simulink model "test"  (R2020a)
settings: Solver=FixedStepAuto  StartTime=0.0  StopTime=inf  FixedStep=.001  RelTol=1e-3  EnableMultiTasking=on
libraries: GPIO_Lib x2, STM32_Config_Lib x1, USART_Lib x1
settings Model: Creator=brunj  LastModifiedBy=tuziz
settings DataIOCC: LimitDataPoints=on  SaveFormat=Array  ReturnWorkspaceOutputs=off
settings OptimizationCC: DefaultParameterBehavior=Inlined  PassReuseOutputArgsAs=Individual arguments  LifeSpan=1  EfficientTunableParamExpr=on
settings DebuggingCC: UnderspecifiedInitializationDetection=Classic  MergeDetectMultiDrivingBlocksExec=none  SolverPrmCheckMsg=warning  AllowSymbolicDim=off  StrictBusMsg=ErrorOnBusTreatedAsVector  SFUnexpectedBacktrackingDiag=warning  SFNoUnconditionalDefaultTransitionDiag=warning  SFUndirectedBroadcastEventsDiag=error  SFExecutionAtInitializationDiag=none  ArithmeticOperatorsInVariantConditions=warning
settings HardwareCC: ProdBitPerPointer=32  ProdBitPerSizeT=32  ProdBitPerPtrDiffT=32  ProdLargestAtomicInteger=Integer  ProdWordSize=32  ProdHWDeviceType=STMicroelectronics->STM32 32-bit Cortex-M
settings ModelReferenceCC: PropagateSignalLabelsOutOfModel=off
settings SFSimCC: SimUseLocalCustomCode=off  CompileTimeRecursionLimit=0  EnableRuntimeRecursion=off  MATLABDynamicMemAlloc=off  CustomCodeUndefinedFunction=UseInterfaceOnly
settings RTWCC: Description=stm32 (Embedded Target)  SystemTargetFile=stm32.tlc  TemplateMakefile=stm32.tmf  RTWUseLocalCustomCode=off  IncludeHyperlinkInReport=on
settings CodeAppCC: IgnoreCustomStorageClasses=off  CustomSymbolStrType=$N$R$M  SimulinkBlockComments=off
settings STFCustomTargetCC: ParMdlRefBuildCompliant=on  IncludeMdlTerminateFcn=off  CombineOutputUpdateFcns=on  ERTCustomFileBanners=on  SupportNonFinite=off  SupportComplex=off  SupportContinuousTime=off  SupportNonInlinedSFcns=off  RemoveResetFunc=on  ParenthesesLevel=Maximum  CastingMode=Standards  MATLABClassNameForMDSCustomization=Simulink.SoftwareTarget.ERTCustomization  SystemTargetFile=stm32.tlc
settings ERTTargetCC: MultiwordLength=2048  CompOptLevelCompliant=off  ConcurrentExecutionCompliant=off  IncludeMdlTerminateFcn=off  SupportNonFinite=off  SupportComplex=off  ParenthesesLevel=Maximum  CastingMode=Standards  ModelStepFunctionPrototypeControlCompliant=off  CPPClassGenCompliant=off  UseToolchainInfoCompliant=off  ExtModeTransport=1  ExtModeStaticAllocSize=256  ExtModeMexArgs=0,1,115200,10  InlinedParameterPlacement=NonHierarchical  ERTSrcFileBannerTemplate=sourceFileTemplate.cgt  ERTHdrFileBannerTemplate=sourceFileTemplate.cgt  ERTDataSrcFileTemplate=sourceFileTemplate.cgt  ERTDataHdrFileTemplate=sourceFileTemplate.cgt  ERTCustomFileTemplate=customRoutineProcess.tlc  ConvertIfToSwitch=off  SuppressUnreachableDefaultCases=off  EnableSignedLeftShifts=off  EnableSignedRightShifts=off
settings ConfigComp: CovMetricSettings=dw  CovHtmlReporting=on  CovSaveCumulativeToWorkspaceVar=on  CovSaveSingleToWorkspaceVar=on  CovExternalEMLEnable=off  CovSFcnEnable=off

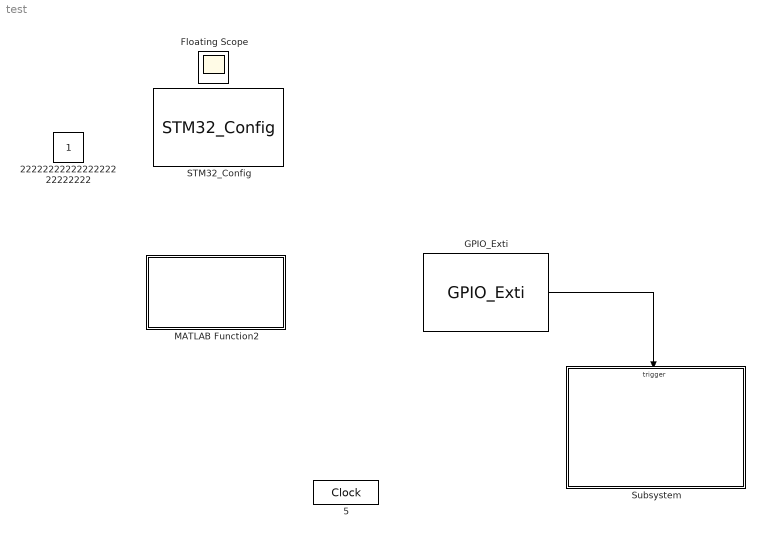
== system test ==
  GPIO_Exti : GPIO_Lib/GPIO_Exti  Port_name=GPIOE  Pin_0=on  Pin_1=off  Pin_2=off  Pin_3=off  Pin_4=off  Pin_5=off  Pin_6=off  Pin_7=off  Pin_8=off  Pin_9=off  Pin_10=off  Pin_11=off  Pin_12=off  Pin_13=off  Pin_14=off  Pin_15=off  PinList=GPIOE0
      settings: SourceProductName=Target Support Package - STM32 Adapter
  MATLAB Function2 : MATLAB Function  Priority=0  TreatAsAtomicUnit=on
  STM32_Config : STM32_Config_Lib/STM32_Config  Priority=0  Project_Path=.\  Config_File=test.ioc  MCU_Name=STM32F407VGTx
      settings: SourceProductName=Target Support Package - STM32 Adapter
  Subsystem : Subsystem
  2222222222222222222222222 : Constant  IOType=siggen
  5 : DigitalClock  IOType=siggen
  Floating Scope : Scope
  wires:
  GPIO_Exti/1 -> Subsystem/Trigger

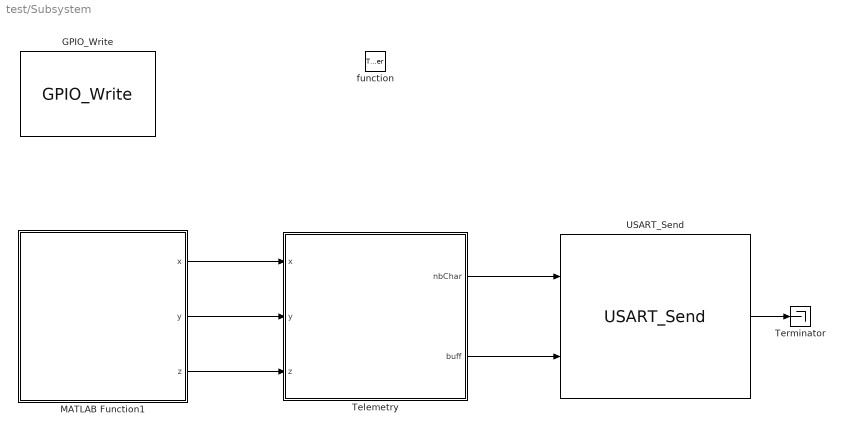
== system test/Subsystem ==
  function : TriggerPort  TriggerType=function-call  VariantControl=Variant
  GPIO_Write : GPIO_Lib/GPIO_Write  Port_name=GPIOD  Pin0=off  Toggle_Pin0=off  Pin1=off  Toggle_Pin1=off  Pin2=off  Toggle_Pin2=off  Pin3=off  Toggle_Pin3=off  Pin4=off  Toggle_Pin4=off  Pin5=off  Toggle_Pin5=off  Pin6=off  Toggle_Pin6=off  Pin7=off  Toggle_Pin7=off  Pin8=off  Toggle_Pin8=off  Pin9=off  Toggle_Pin9=off  Pin10=off  Toggle_Pin10=off  Pin11=off  Toggle_Pin11=off  Pin12=on  Toggle_Pin12=on  Pin13=off  Toggle_Pin13=off  Pin14=off  Toggle_Pin14=off  Pin15=off  Toggle_Pin15=off  PinList="GPIOD12  13  14  15GPIOE3"
      settings: SourceProductName=Target Support Package - STM32 Adapter
  MATLAB Function1 : MATLAB Function  Priority=0  TreatAsAtomicUnit=on
  Telemetry : MATLAB Function  TreatAsAtomicUnit=on
  Terminator : Terminator
  USART_Send : USART_Lib/USART_Send  USART_name=USART3  Buff_size=22  nbUsart=1  usartMode=Asynchronous  usartDma_Rx=off  usartDma_Tx=off  usartIt=on
      settings: SourceProductName=Target Support Package - STM32 Adapter
  wires:
  USART_Send/1 -> Terminator/1
  MATLAB Function1/2(y) -> Telemetry/2(y)
  Telemetry/1(nbChar) -> USART_Send/1
  Telemetry/2(buff) -> USART_Send/2
  MATLAB Function1/1(x) -> Telemetry/1(x)
  MATLAB Function1/3(z) -> Telemetry/3(z)

== matlab function test/MATLAB Function2 ==
function LIS302_Init()
if coder.target('Sfun')
    % Executing in MATLAB, Buff is null
else
    coder.cinclude('LIS3DSH.h');
    
    % Executing in the generated code.
    coder.ceval('accelInit');  
end

== matlab function test/Subsystem/Telemetry ==
  data: x input; nbChar output uint16 size=1; buff output uint32 size=1; y input; z input
function [nbChar, buff] = convert(x,y,z)
if coder.target('Sfun')
    % Executing in MATLAB, Buff is null
    buff = uint32(0);
    nbChar = uint16(0);
else
    coder.cinclude('stdio.h');
    coder.cinclude('main.h');
    coder.cinclude('string.h')
    coder.cinclude('getBuffPtr.h');

    % Executing in the generated code.
    string = char(zeros(1,22));
    stringSize = uint16(size(string,2));
    stringFormat = char(['%6i,','%6i,','%6i',10,13,0]);
    coder.ceval('snprintf',coder.wref(string),stringSize,coder.rref(stringFormat),x,y,z);
    buff = coder.ceval('getBuffPtr',coder.rref(string));
    nbChar = coder.ceval('strlen',string);
end
end

== matlab function test/Subsystem/MATLAB Function1 ==
  data: x output; y output; z output
function [x,y,z]= read_accel()
if coder.target('Sfun')
    % Executing in MATLAB, Buff is null
    x = int16(0);
    y = int16(0);
    z = int16(0);
else
    coder.cinclude('LIS3DSH.h');
    
    % Executing in the generated code.
    coder.ceval('read_accel');  
    
    x = coder.ceval('accel_X');    
    y = coder.ceval('accel_Y'); 
    z = coder.ceval('accel_Z'); 
end
